simulink model "KalmanLTI"  (Simulink 7.0)
settings: Solver=FixedStepDiscrete  StartTime=0.0  StopTime=10.0  RelTol=1e-3
values from neighbouring files (symbols this model uses):
  A = [0.8110   -0.0348    0.0499    0.3313 ... (first row only)    [feedbackviewKF.m]
  A1 = A    (= 0)    [feedbackviewKF.m]
  B = [-0.0130    0.0024 ... (first row only)    [feedbackviewKF.m]
  B1 = B    (= 1)    [feedbackviewKF.m]
  C = [0.1685   -0.9595   -0.0755   -0.3771 ... (first row only)    [feedbackviewKF.m]
  C1 = C    (= 1)    [feedbackviewKF.m]
  D = [0 0;0 0]    [feedbackviewKF.m]
  D1 = D    (= 0)    [feedbackviewKF.m]
  K = y(:,:,end)    [feedbackviewKF.m]
  Q = diag([0.5^2 0.2^2 0.3^2 0.5^2])    [feedbackviewKF.m]
  R = eye(2)    [feedbackviewKF.m]
  x0 = randn(4,1)    [feedbackviewKF.m]
  x1 = zeros(4,1)    [feedbackviewKF.m]
settings Model: Creator=fo1521  LastModifiedBy=fo1521
settings DebuggingCC: SaveWithParameterizedLinksMsg=none  MultiTaskCondExecSysMsg=none  StrictBusMsg=None
settings HardwareCC: TargetHWDeviceType=32-bit Generic
settings RTWCC: IncludeERTFirstTime=on
settings GRTTargetCC: TargetFcnLib=ansi_tfl_tmw.mat

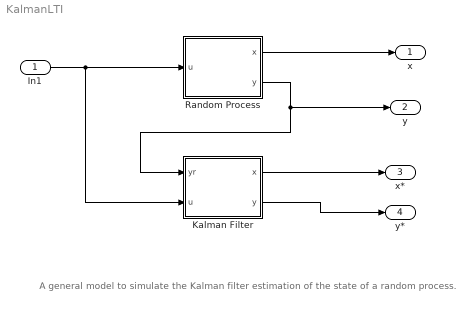
== system KalmanLTI ==
  note: A general model to simulate the Kalman filter estimation of the state of a random process.
  In1 : Inport  OutDataType=sfix(16)  OutScaling=2^0
  Kalman Filter : Subsystem  mask{x0=x1, A=A1, B=B1, C=C1, D=D1, K=K}
      mask help:
      | Linear Random Process
      | x(k+1)=Ax(k)+Bu(k)+w
      | y(k)=Cx(k)+Du(k)+v
      | w~N(0,Q)
      | w~N(0,R)
      mask Display:
      | disp(sprintf('Kalman\n Filter'))
      | port_label('output',2,'y')
      | port_label('output',1,'x')
      | port_label('input',1,'y')
      | port_label('input',2,'u')
  Random Process : Subsystem  mask{x0=x0, A=A, B=B, C=C, D=D, Q=sqrt(Q), R=sqrt(R)}
      mask help:
      | Linear Random Process
      | x(k+1)=Ax(k)+Bu(k)+w
      | y(k)=Cx(k)+Du(k)+v
      | w~N(0,Q)
      | w~N(0,R)
      mask Display:
      | disp(sprintf('Linear\n Random\n System'))
      | port_label('output',1,'x')
      | port_label('output',2,'y')
      | port_label('input',1,'u')
  x : Outport  OutDataType=sfix(16)  OutScaling=2^0
  y : Outport  Port=2  OutDataType=sfix(16)  OutScaling=2^0
  x* : Outport  Port=3  OutDataType=sfix(16)  OutScaling=2^0
  y* : Outport  Port=4  OutDataType=sfix(16)  OutScaling=2^0
  wires:
  Random Process/2(y) -> y/1, Kalman Filter/1(yr)
  In1/1 -> Random Process/1(u), Kalman Filter/2(u)
  Random Process/1(x) -> x/1
  Kalman Filter/1(x) -> x*/1
  Kalman Filter/2(y) -> y*/1

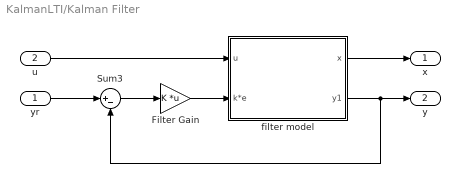
== system KalmanLTI/Kalman Filter ==
  yr : Inport  OutDataType=sfix(16)  OutScaling=2^0
  u : Inport  Port=2  PortDimensions=size(B,2)  OutDataType=sfix(16)  OutScaling=2^0
  Filter Gain : Gain  Gain=K  Multiplication=Matrix(K*u)  ParameterDataType=sfix(16)  ParameterScaling=2^0  OutDataType=sfix(16)  OutScaling=2^0
  Sum3 : Sum  Inputs=|+-  OutDataType=sfix(16)  OutScaling=2^0
  filter model : Subsystem
  x : Outport  OutDataType=sfix(16)  OutScaling=2^0
  y : Outport  Port=2  OutDataType=sfix(16)  OutScaling=2^0
  wires:
  u/1 -> filter model/1(u)
  filter model/1(x) -> x/1
  filter model/2(y1) -> y/1, Sum3/2
  Sum3/1 -> Filter Gain/1
  yr/1 -> Sum3/1
  Filter Gain/1 -> filter model/2(k*e)

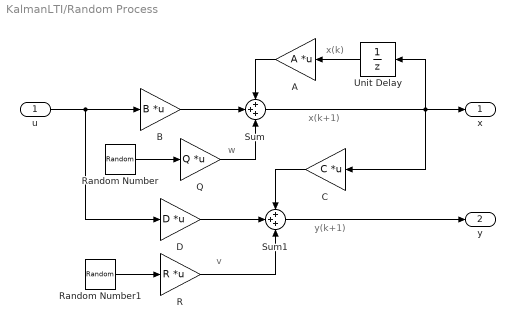
== system KalmanLTI/Random Process ==
  note: x(k+1)
  note: y(k+1)
  note: x(k)
  note: w
  note: v
  u : Inport  PortDimensions=size(B,2)  OutDataType=sfix(16)  OutScaling=2^0
  A : Gain  Orientation=left  Gain=A  Multiplication=Matrix(K*u)  ParameterDataType=sfix(16)  ParameterScaling=2^0  OutDataType=sfix(16)  OutScaling=2^0
  B : Gain  Gain=B  Multiplication=Matrix(K*u)  ParameterDataType=sfix(16)  ParameterScaling=2^0  OutDataType=sfix(16)  OutScaling=2^0
  C : Gain  Orientation=left  Gain=C  Multiplication=Matrix(K*u)  ParameterDataType=sfix(16)  ParameterScaling=2^0  OutDataType=sfix(16)  OutScaling=2^0
  D : Gain  Gain=D  Multiplication=Matrix(K*u)  ParameterDataType=sfix(16)  ParameterScaling=2^0  OutDataType=sfix(16)  OutScaling=2^0
  Q : Gain  Gain=Q  Multiplication=Matrix(K*u)  ParameterDataType=sfix(16)  ParameterScaling=2^0  OutDataType=sfix(16)  OutScaling=2^0
  R : Gain  Gain=R  Multiplication=Matrix(K*u)  ParameterDataType=sfix(16)  ParameterScaling=2^0  OutDataType=sfix(16)  OutScaling=2^0
  Random Number : RandomNumber  Mean=zeros(size(Q,1),1)  Variance=ones(size(Q,1),1)  Seed=7  SampleTime=1
  Random Number1 : RandomNumber  Mean=zeros(size(R,1),1)  Variance=ones(size(R,1),1)  SampleTime=1
  Sum : Sum  Inputs=+++  OutDataType=sfix(16)  OutScaling=2^0
  Sum1 : Sum  Inputs=+++  OutDataType=sfix(16)  OutScaling=2^0
  Unit Delay : UnitDelay  Orientation=left  X0=x0
  x : Outport  OutDataType=sfix(16)  OutScaling=2^0
  y : Outport  Port=2  OutDataType=sfix(16)  OutScaling=2^0
  wires:
  u/1 -> B/1, D/1
  Random Number/1 -> Q/1
  B/1 -> Sum/2
  C/1 -> Sum1/1
  D/1 -> Sum1/2
  Random Number1/1 -> R/1
  R/1 -> Sum1/3
  Sum1/1 -> y/1
  Sum/1 -> Unit Delay/1, x/1, C/1
  Unit Delay/1 -> A/1
  A/1 -> Sum/1
  Q/1 -> Sum/3

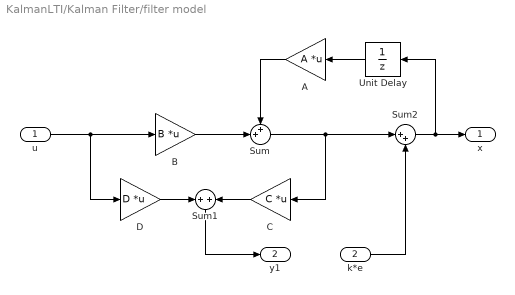
== system KalmanLTI/Kalman Filter/filter model ==
  u : Inport  PortDimensions=size(B,2)  OutDataType=sfix(16)  OutScaling=2^0
  k*e : Inport  Port=2  OutDataType=sfix(16)  OutScaling=2^0
  A : Gain  Orientation=left  Gain=A  Multiplication=Matrix(K*u)  ParameterDataType=sfix(16)  ParameterScaling=2^0  OutDataType=sfix(16)  OutScaling=2^0
  B : Gain  Gain=B  Multiplication=Matrix(K*u)  ParameterDataType=sfix(16)  ParameterScaling=2^0  OutDataType=sfix(16)  OutScaling=2^0
  C : Gain  Orientation=left  Gain=C  Multiplication=Matrix(K*u)  ParameterDataType=sfix(16)  ParameterScaling=2^0  OutDataType=sfix(16)  OutScaling=2^0
  D : Gain  Gain=D  Multiplication=Matrix(K*u)  ParameterDataType=sfix(16)  ParameterScaling=2^0  OutDataType=sfix(16)  OutScaling=2^0
  Sum : Sum  Inputs=++|  OutDataType=sfix(16)  OutScaling=2^0
  Sum1 : Sum  Orientation=down  Inputs=+|+  OutDataType=sfix(16)  OutScaling=2^0
  Sum2 : Sum  Inputs=|++  OutDataType=sfix(16)  OutScaling=2^0
  Unit Delay : UnitDelay  Orientation=left  X0=x0
  x : Outport  OutDataType=sfix(16)  OutScaling=2^0
  y1 : Outport  Port=2  OutDataType=sfix(16)  OutScaling=2^0
  wires:
  u/1 -> B/1, D/1
  B/1 -> Sum/2
  A/1 -> Sum/1
  Unit Delay/1 -> A/1
  Sum/1 -> Sum2/1, C/1
  Sum2/1 -> x/1, Unit Delay/1
  D/1 -> Sum1/1
  C/1 -> Sum1/2
  k*e/1 -> Sum2/2
  Sum1/1 -> y1/1
